simulink model "xaui_switch"  (Simulink 7.4)
settings: Solver=ode45  StartTime=0.0  StopTime=100  RelTol=1e-3
undefined symbols (not defined in the file): ROACH
libraries: xbsIndex_r4 x22, xps_library x10
settings Model: Creator=wjm  LastModifiedBy=wjm
settings OptimizationCC: InitFltsAndDblsToZero=on

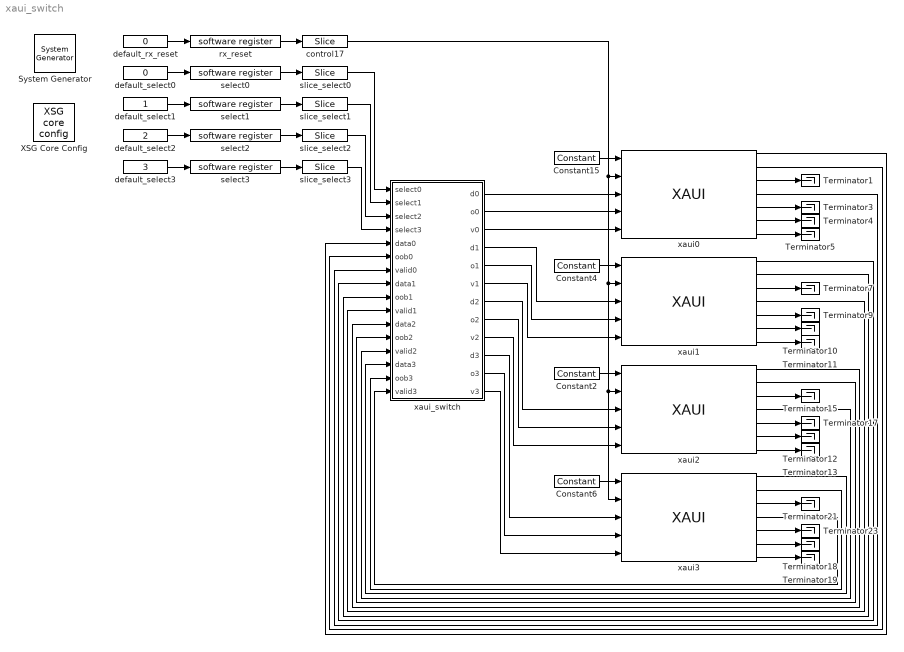
== system xaui_switch ==
  " System Generator" : xbsIndex_r4/ System Generator  Tag=genX  SystemSampleTime=-1  xilinxfamily=virtex5  part=xc5vsx95t  speed=-1  package=ff1136  synthesis_tool=XST  clock_wrapper=Clock Enables  directory=./xaui_loop/sysgen  testbench=off  simulink_period=1  sysclk_period=5  dcm_input_clock_period=100  incr_netlist=off  trim_vbits=Everywhere in SubSystem  dbl_ovrd=According to Block Masks  core_generation=According to Block Masks  run_coregen=off  deprecated_control=off  eval_field=0  block_type=sysgen
      settings: block_version=10.1.1
  Constant{2,4,6,15} (4 alike) : xbsIndex_r4/Constant  arith_type=Boolean  const=1  n_bits=1  bin_pt=0  explicit_period=on  period=1  equ=P=C  opselect=C  inp2=PCIN>>17  opr=+  inp1=P  carry=CIN  dbl_ovrd=off  block_type=constant
      settings: block_version=10.1.1
  Terminator{1,3..5,7,9..13,15,17..19,21,23} (16 alike) : Terminator
  XSG Core Config : xps_library/XSG core config  Tag=xps:xsg  SystemSampleTime=-1  hw_sys=ROACH:sx95t  ibob_linux=off  clk_src=sys_clk2x  iBOB_clk_src=sys_clk2x  BEE2_ctrl_clk_src=sys_clk  BEE2_usr_clk_src=sys_clk2x  ROACH_clk_src=sys_clk2x  CORR_clk_src=sys_clk  gpio_clk_io_group=iBOB:sma  gpio_clk_bit_index=0  clk_rate=200  sample_period=1  synthesis_tool=XST  mpc_type=powerpc440_ext
  control17 : xbsIndex_r4/Slice  nbits=1  boolean_output=on  mode=Lower Bit Location + Width  bit1=0  base1=MSB of Input  bit0=0  base0=LSB of Input  dbl_ovrd=off  block_type=slice
      settings: infoedit="Extracts a given range of bits from each input sample and presents it at the output.  The output type is ordinarily unsigned with binary point at zero, but can be Boolean when the slice is one bit wide.<P><P>Hardware notes: In hardware this block costs nothing."  block_version=10.1.3
  default_rx_reset : Constant  Value=0  OutDataType=sfix(16)  OutScaling=2^0  SampleTime=1
  default_select0 : Constant  Value=0  OutDataType=sfix(16)  OutScaling=2^0  SampleTime=1
  default_select1 : Constant  OutDataType=sfix(16)  OutScaling=2^0  SampleTime=1
  default_select2 : Constant  Value=2  OutDataType=sfix(16)  OutScaling=2^0  SampleTime=1
  default_select3 : Constant  Value=3  OutDataType=sfix(16)  OutScaling=2^0  SampleTime=1
  rx_reset : xps_library/software register  Tag=xps:sw_reg  SystemSampleTime=-1  io_dir=From Processor  arith_type=Unsigned  bitwidth=32  bin_pt=0  sample_period=1  gw_name=xaui_switch_rx_reset_user_data_out
  select{0..3} (4 alike) : xps_library/software register  Tag=xps:sw_reg  SystemSampleTime=-1  io_dir=From Processor  arith_type=Unsigned  bitwidth=32  bin_pt=0  sample_period=1  gw_name=xaui_switch_rx_reset_user_data_out
  slice_select{0..3} (4 alike) : xbsIndex_r4/Slice  nbits=2  boolean_output=off  mode=Lower Bit Location + Width  bit1=0  base1=MSB of Input  bit0=0  base0=LSB of Input  dbl_ovrd=off  block_type=slice
      settings: block_version=10.1.3
  xaui0 : xps_library/XAUI  Tag=xps:xaui  SystemSampleTime=-1  demux=1  port=ROACH:0  open_phy=on  show_param=off  pre_emph=3  swing=800
  xaui1 : xps_library/XAUI  Tag=xps:xaui  SystemSampleTime=-1  demux=1  port=ROACH:1  open_phy=on  show_param=off  pre_emph=3  swing=800
  xaui2 : xps_library/XAUI  Tag=xps:xaui  SystemSampleTime=-1  demux=1  port=ROACH:2  open_phy=on  show_param=off  pre_emph=3  swing=800
  xaui3 : xps_library/XAUI  Tag=xps:xaui  SystemSampleTime=-1  demux=1  port=ROACH:3  open_phy=on  show_param=off  pre_emph=3  swing=800
  xaui_switch : Subsystem
  wires:
  Constant15/1 -> xaui0/1
  Constant4/1 -> xaui1/1
  default_rx_reset/1 -> rx_reset/1
  rx_reset/1 -> control17/1
  control17/1 -> xaui0/2, xaui1/2, xaui2/2, xaui3/2
  Constant2/1 -> xaui2/1
  Constant6/1 -> xaui3/1
  xaui3/3 -> Terminator21/1
  xaui3/5 -> Terminator23/1
  xaui3/6 -> Terminator18/1
  xaui3/7 -> Terminator19/1
  xaui2/3 -> Terminator15/1
  xaui2/5 -> Terminator17/1
  xaui2/6 -> Terminator12/1
  xaui2/7 -> Terminator13/1
  xaui1/3 -> Terminator7/1
  xaui1/5 -> Terminator9/1
  xaui1/6 -> Terminator10/1
  xaui1/7 -> Terminator11/1
  xaui0/3 -> Terminator1/1
  xaui0/5 -> Terminator3/1
  xaui0/6 -> Terminator4/1
  xaui0/7 -> Terminator5/1
  default_select0/1 -> select0/1
  select0/1 -> slice_select0/1
  default_select1/1 -> select1/1
  select1/1 -> slice_select1/1
  default_select2/1 -> select2/1
  select2/1 -> slice_select2/1
  default_select3/1 -> select3/1
  select3/1 -> slice_select3/1
  slice_select0/1 -> xaui_switch/1(select0)
  slice_select1/1 -> xaui_switch/2(select1)
  slice_select2/1 -> xaui_switch/3(select2)
  slice_select3/1 -> xaui_switch/4(select3)
  xaui_switch/1(d0) -> xaui0/3
  xaui_switch/2(o0) -> xaui0/4
  xaui_switch/3(v0) -> xaui0/5
  xaui_switch/4(d1) -> xaui1/3
  xaui_switch/5(o1) -> xaui1/4
  xaui_switch/6(v1) -> xaui1/5
  xaui_switch/7(d2) -> xaui2/3
  xaui_switch/8(o2) -> xaui2/4
  xaui_switch/9(v2) -> xaui2/5
  xaui_switch/10(d3) -> xaui3/3
  xaui_switch/11(o3) -> xaui3/4
  xaui_switch/12(v3) -> xaui3/5
  xaui0/1 -> xaui_switch/5(data0)
  xaui0/2 -> xaui_switch/6(oob0)
  xaui0/4 -> xaui_switch/7(valid0)
  xaui1/1 -> xaui_switch/8(data1)
  xaui1/2 -> xaui_switch/9(oob1)
  xaui1/4 -> xaui_switch/10(valid1)
  xaui2/1 -> xaui_switch/11(data2)
  xaui2/2 -> xaui_switch/12(oob2)
  xaui2/4 -> xaui_switch/13(valid2)
  xaui3/1 -> xaui_switch/14(data3)
  xaui3/2 -> xaui_switch/15(oob3)
  xaui3/4 -> xaui_switch/16(valid3)

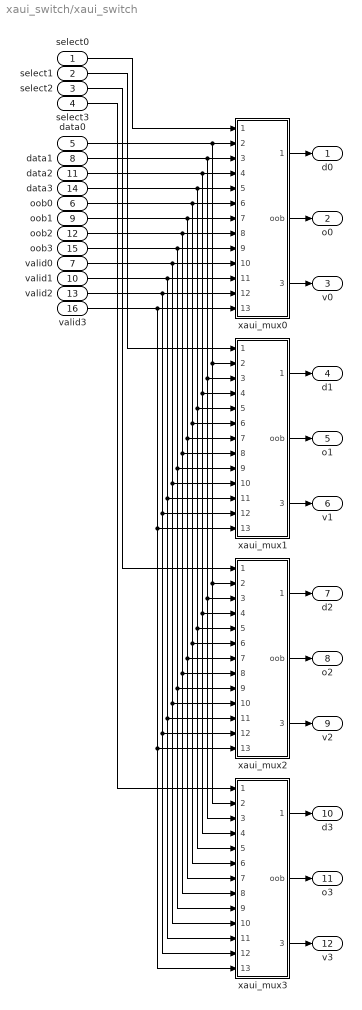
== system xaui_switch/xaui_switch ==
  select0 : Inport
  select1 : Inport  Port=2
  select2 : Inport  Port=3
  select3 : Inport  Port=4
  data0 : Inport  Port=5
  oob0 : Inport  Port=6
  valid0 : Inport  Port=7
  data1 : Inport  Port=8
  oob1 : Inport  Port=9
  valid1 : Inport  Port=10
  data2 : Inport  Port=11
  oob2 : Inport  Port=12
  valid2 : Inport  Port=13
  data3 : Inport  Port=14
  oob3 : Inport  Port=15
  valid3 : Inport  Port=16
  xaui_mux0 : Subsystem
  xaui_mux1 : Subsystem
  xaui_mux2 : Subsystem
  xaui_mux3 : Subsystem
  d0 : Outport
  o0 : Outport  Port=2
  v0 : Outport  Port=3
  d1 : Outport  Port=4
  o1 : Outport  Port=5
  v1 : Outport  Port=6
  d2 : Outport  Port=7
  o2 : Outport  Port=8
  v2 : Outport  Port=9
  d3 : Outport  Port=10
  o3 : Outport  Port=11
  v3 : Outport  Port=12
  wires:
  xaui_mux0/1(data) -> d0/1
  xaui_mux0/2(oob) -> o0/1
  xaui_mux0/3(valid) -> v0/1
  xaui_mux1/1(data) -> d1/1
  xaui_mux1/2(oob) -> o1/1
  xaui_mux1/3(valid) -> v1/1
  xaui_mux2/1(data) -> d2/1
  xaui_mux2/2(oob) -> o2/1
  xaui_mux2/3(valid) -> v2/1
  xaui_mux3/1(data) -> d3/1
  xaui_mux3/2(oob) -> o3/1
  xaui_mux3/3(valid) -> v3/1
  select0/1 -> xaui_mux0/1(select)
  data0/1 -> xaui_mux0/2(data0), xaui_mux1/2(data0), xaui_mux3/2(data0), xaui_mux2/2(data0)
  data1/1 -> xaui_mux0/3(data1), xaui_mux1/3(data1), xaui_mux3/3(data1), xaui_mux2/3(data1)
  data2/1 -> xaui_mux0/4(data2), xaui_mux1/4(data2), xaui_mux3/4(data2), xaui_mux2/4(data2)
  data3/1 -> xaui_mux0/5(data3), xaui_mux1/5(data3), xaui_mux3/5(data3), xaui_mux2/5(data3)
  oob0/1 -> xaui_mux0/6(oob0), xaui_mux1/6(oob0), xaui_mux3/6(oob0), xaui_mux2/6(oob0)
  oob1/1 -> xaui_mux0/7(oob1), xaui_mux1/7(oob1), xaui_mux3/7(oob1), xaui_mux2/7(oob1)
  oob2/1 -> xaui_mux0/8(oob2), xaui_mux1/8(oob2), xaui_mux3/8(oob2), xaui_mux2/8(oob2)
  oob3/1 -> xaui_mux0/9(oob3), xaui_mux1/9(oob3), xaui_mux3/9(oob3), xaui_mux2/9(oob3)
  valid0/1 -> xaui_mux0/10(valid0), xaui_mux1/10(valid0), xaui_mux3/10(valid0), xaui_mux2/10(valid0)
  valid1/1 -> xaui_mux0/11(valid1), xaui_mux1/11(valid1), xaui_mux3/11(valid1), xaui_mux2/11(valid1)
  valid2/1 -> xaui_mux0/12(valid2), xaui_mux1/12(valid2), xaui_mux3/12(valid2), xaui_mux2/12(valid2)
  valid3/1 -> xaui_mux0/13(valid3), xaui_mux1/13(valid3), xaui_mux3/13(valid3), xaui_mux2/13(valid3)
  select1/1 -> xaui_mux1/1(select)
  select2/1 -> xaui_mux2/1(select)
  select3/1 -> xaui_mux3/1(select)

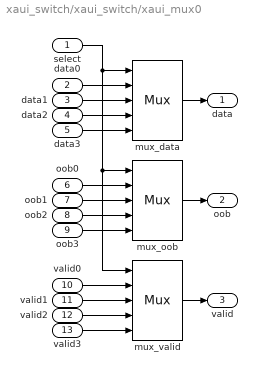
== system xaui_switch/xaui_switch/xaui_mux0 ==
  select : Inport
  data0 : Inport  Port=2
  data1 : Inport  Port=3
  data2 : Inport  Port=4
  data3 : Inport  Port=5
  oob0 : Inport  Port=6
  oob1 : Inport  Port=7
  oob2 : Inport  Port=8
  oob3 : Inport  Port=9
  valid0 : Inport  Port=10
  valid1 : Inport  Port=11
  valid2 : Inport  Port=12
  valid3 : Inport  Port=13
  mux_data : xbsIndex_r4/Mux  inputs=4  en=off  latency=3  precision=Full  arith_type=Unsigned  n_bits=16  bin_pt=14  quantization=Truncate  overflow=Wrap  dbl_ovrd=off  block_type=mux
      settings: block_version=11.4
  mux_oob : xbsIndex_r4/Mux  inputs=4  en=off  latency=3  precision=Full  arith_type=Unsigned  n_bits=16  bin_pt=14  quantization=Truncate  overflow=Wrap  dbl_ovrd=off  block_type=mux
      settings: block_version=11.4
  mux_valid : xbsIndex_r4/Mux  inputs=4  en=off  latency=3  precision=Full  arith_type=Unsigned  n_bits=16  bin_pt=14  quantization=Truncate  overflow=Wrap  dbl_ovrd=off  block_type=mux
      settings: block_version=11.4
  data : Outport
  oob : Outport  Port=2
  valid : Outport  Port=3
  wires:
  data0/1 -> mux_data/2
  data1/1 -> mux_data/3
  mux_data/1 -> data/1
  data2/1 -> mux_data/4
  data3/1 -> mux_data/5
  oob0/1 -> mux_oob/2
  oob1/1 -> mux_oob/3
  mux_oob/1 -> oob/1
  oob2/1 -> mux_oob/4
  oob3/1 -> mux_oob/5
  valid0/1 -> mux_valid/2
  valid1/1 -> mux_valid/3
  valid2/1 -> mux_valid/4
  valid3/1 -> mux_valid/5
  mux_valid/1 -> valid/1
  select/1 -> mux_data/1, mux_valid/1, mux_oob/1

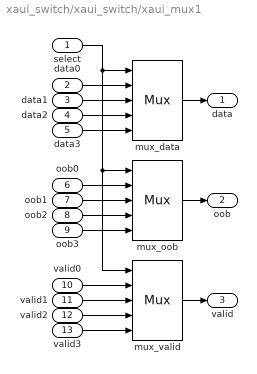
== system xaui_switch/xaui_switch/xaui_mux1 ==
  select : Inport
  data0 : Inport  Port=2
  data1 : Inport  Port=3
  data2 : Inport  Port=4
  data3 : Inport  Port=5
  oob0 : Inport  Port=6
  oob1 : Inport  Port=7
  oob2 : Inport  Port=8
  oob3 : Inport  Port=9
  valid0 : Inport  Port=10
  valid1 : Inport  Port=11
  valid2 : Inport  Port=12
  valid3 : Inport  Port=13
  mux_data : xbsIndex_r4/Mux  inputs=4  en=off  latency=3  precision=Full  arith_type=Unsigned  n_bits=16  bin_pt=14  quantization=Truncate  overflow=Wrap  dbl_ovrd=off  block_type=mux
      settings: block_version=11.4
  mux_oob : xbsIndex_r4/Mux  inputs=4  en=off  latency=3  precision=Full  arith_type=Unsigned  n_bits=16  bin_pt=14  quantization=Truncate  overflow=Wrap  dbl_ovrd=off  block_type=mux
      settings: block_version=11.4
  mux_valid : xbsIndex_r4/Mux  inputs=4  en=off  latency=3  precision=Full  arith_type=Unsigned  n_bits=16  bin_pt=14  quantization=Truncate  overflow=Wrap  dbl_ovrd=off  block_type=mux
      settings: block_version=11.4
  data : Outport
  oob : Outport  Port=2
  valid : Outport  Port=3
  wires:
  select/1 -> mux_oob/1, mux_valid/1, mux_data/1
  mux_valid/1 -> valid/1
  valid3/1 -> mux_valid/5
  valid2/1 -> mux_valid/4
  valid1/1 -> mux_valid/3
  valid0/1 -> mux_valid/2
  oob3/1 -> mux_oob/5
  oob2/1 -> mux_oob/4
  mux_oob/1 -> oob/1
  oob1/1 -> mux_oob/3
  oob0/1 -> mux_oob/2
  data3/1 -> mux_data/5
  data2/1 -> mux_data/4
  mux_data/1 -> data/1
  data1/1 -> mux_data/3
  data0/1 -> mux_data/2

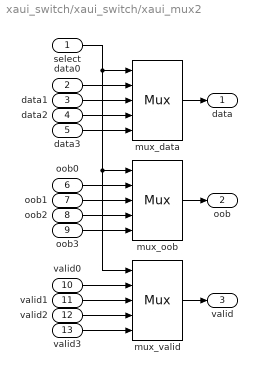
== system xaui_switch/xaui_switch/xaui_mux2 ==
  select : Inport
  data0 : Inport  Port=2
  data1 : Inport  Port=3
  data2 : Inport  Port=4
  data3 : Inport  Port=5
  oob0 : Inport  Port=6
  oob1 : Inport  Port=7
  oob2 : Inport  Port=8
  oob3 : Inport  Port=9
  valid0 : Inport  Port=10
  valid1 : Inport  Port=11
  valid2 : Inport  Port=12
  valid3 : Inport  Port=13
  mux_data : xbsIndex_r4/Mux  inputs=4  en=off  latency=3  precision=Full  arith_type=Unsigned  n_bits=16  bin_pt=14  quantization=Truncate  overflow=Wrap  dbl_ovrd=off  block_type=mux
      settings: block_version=11.4
  mux_oob : xbsIndex_r4/Mux  inputs=4  en=off  latency=3  precision=Full  arith_type=Unsigned  n_bits=16  bin_pt=14  quantization=Truncate  overflow=Wrap  dbl_ovrd=off  block_type=mux
      settings: block_version=11.4
  mux_valid : xbsIndex_r4/Mux  inputs=4  en=off  latency=3  precision=Full  arith_type=Unsigned  n_bits=16  bin_pt=14  quantization=Truncate  overflow=Wrap  dbl_ovrd=off  block_type=mux
      settings: block_version=11.4
  data : Outport
  oob : Outport  Port=2
  valid : Outport  Port=3
  wires:
  data0/1 -> mux_data/2
  data1/1 -> mux_data/3
  mux_data/1 -> data/1
  data2/1 -> mux_data/4
  data3/1 -> mux_data/5
  oob0/1 -> mux_oob/2
  oob1/1 -> mux_oob/3
  mux_oob/1 -> oob/1
  oob2/1 -> mux_oob/4
  oob3/1 -> mux_oob/5
  valid0/1 -> mux_valid/2
  valid1/1 -> mux_valid/3
  valid2/1 -> mux_valid/4
  valid3/1 -> mux_valid/5
  mux_valid/1 -> valid/1
  select/1 -> mux_data/1, mux_valid/1, mux_oob/1

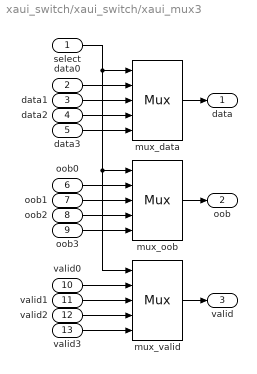
== system xaui_switch/xaui_switch/xaui_mux3 ==
  select : Inport
  data0 : Inport  Port=2
  data1 : Inport  Port=3
  data2 : Inport  Port=4
  data3 : Inport  Port=5
  oob0 : Inport  Port=6
  oob1 : Inport  Port=7
  oob2 : Inport  Port=8
  oob3 : Inport  Port=9
  valid0 : Inport  Port=10
  valid1 : Inport  Port=11
  valid2 : Inport  Port=12
  valid3 : Inport  Port=13
  mux_data : xbsIndex_r4/Mux  inputs=4  en=off  latency=3  precision=Full  arith_type=Unsigned  n_bits=16  bin_pt=14  quantization=Truncate  overflow=Wrap  dbl_ovrd=off  block_type=mux
      settings: block_version=11.4
  mux_oob : xbsIndex_r4/Mux  inputs=4  en=off  latency=3  precision=Full  arith_type=Unsigned  n_bits=16  bin_pt=14  quantization=Truncate  overflow=Wrap  dbl_ovrd=off  block_type=mux
      settings: block_version=11.4
  mux_valid : xbsIndex_r4/Mux  inputs=4  en=off  latency=3  precision=Full  arith_type=Unsigned  n_bits=16  bin_pt=14  quantization=Truncate  overflow=Wrap  dbl_ovrd=off  block_type=mux
      settings: block_version=11.4
  data : Outport
  oob : Outport  Port=2
  valid : Outport  Port=3
  wires:
  select/1 -> mux_oob/1, mux_valid/1, mux_data/1
  mux_valid/1 -> valid/1
  valid3/1 -> mux_valid/5
  valid2/1 -> mux_valid/4
  valid1/1 -> mux_valid/3
  valid0/1 -> mux_valid/2
  oob3/1 -> mux_oob/5
  oob2/1 -> mux_oob/4
  mux_oob/1 -> oob/1
  oob1/1 -> mux_oob/3
  oob0/1 -> mux_oob/2
  data3/1 -> mux_data/5
  data2/1 -> mux_data/4
  mux_data/1 -> data/1
  data1/1 -> mux_data/3
  data0/1 -> mux_data/2
